simulink model "SistemaFunivia"  (R2023b)
settings: Solver=VariableStepAuto  StartTime=0.0  StopTime=100  FixedStep=1e-5
values from neighbouring files (symbols this model uses):
  dq_0 = [0; 0]    [Parametri.m]
  encoder_params = [r, encoder_accuracy, encoder_resolution, encoder_sample_rates]    [Parametri.m]
  encoder_resolution = 2*pi/1200    (= 0.00523598775598)    [Parametri.m]
  F_0 = 1500    [Parametri.m]
  L = 2.2    [Parametri.m]
  l = L - 1.2    (= 1)    [Parametri.m]
  laserd1_params = [laserd1_sample_rates, laserd1_resolution, laserd1_accuracy]    [Parametri.m]
  laserD_params = [laserD_sample_rates, laserD_resolution, laserD_accuracy]    [Parametri.m]
  min_sample_rates = max(sample_rates)    [Parametri.m]
  params = [m, c_a, J, L, l, h, r, g]    [Parametri.m]
  q_0 = [0; -pi/6]    [Parametri.m]
  q_hat_0 = [ dq_0(1) + normrnd(0, 0.1) ... (first row only)    [Parametri.m]
  R_k = diag([(laserD_accuracy/1000)^2, (laserd1_accuracy/1000)^2, (encoder_accuracy/encoder_sample_rates)^2])    [Parametri.m]
libraries: simulink x6, dspswit3 x1, embmathops x1
settings Model: Creator=lucag  LastModifiedBy=edoca

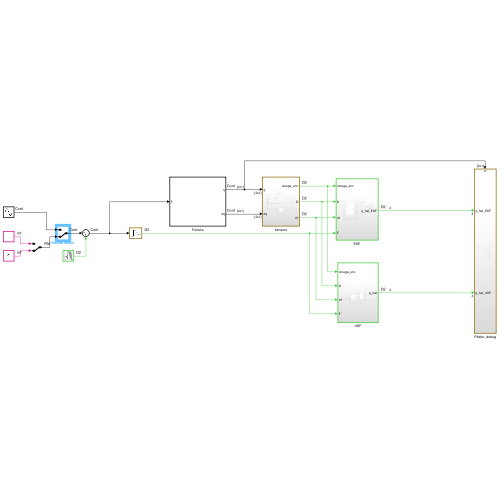
[thumbnail: Simulink's stored preview of the top-level diagram]
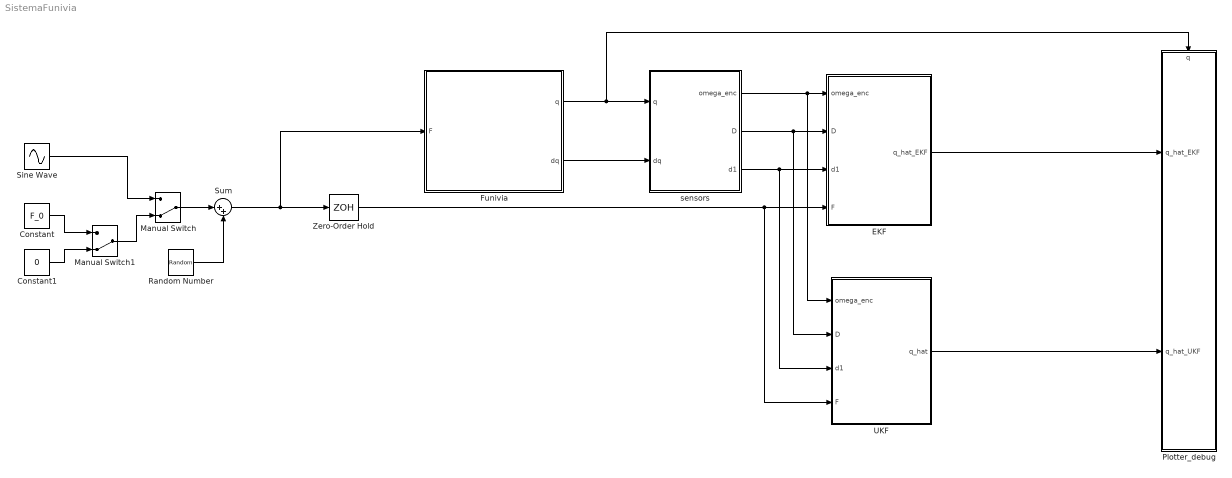
== system SistemaFunivia ==
  Constant : Constant  Value=F_0
  Constant1 : Constant  Value=0
  EKF : Subsystem
  Funivia : Subsystem
  Manual Switch : ManualSwitch  CurrentSetting=0
  Manual Switch1 : ManualSwitch  CurrentSetting=0
  Plotter_debug : Subsystem
      settings: PortSchema="{\"entries\":[{\"content\":{\"sides\":[{\"content\":{\"connectorIds\":[\"In1\",\"In2\"]},\"type\":\"ConnectorPlacement.EquallySpacedRectSide\",\"uuid\":\"d01a7d39-b326-48f3-bf6d-774b593ab054\"},{\"content\":{\"side\":\"RIGHT\"},\"type\":\"ConnectorPlacement.EquallySpacedRectSide\",\"uuid\":\"87cbfa34-b37b-41ae-99cb-fc2d681c6b8e\"},{\"content\":{\"connectorIds\":[\"In3\"],\"side\":\"TOP\"},\"type\":\"ConnectorPlacement.EquallySpacedRectSide\",\"uuid\":\"574a8c95-5b26-494e-b43d-53eefa443978\"}]},\"type\":\"ConnectorPlacement.EquallySpacedConnector\",\"uuid\":\"03fd7438-2859-47c7-88d3-b9f2a0aea320\"}],\"packageUris\":[\"http://schema.mathworks.com/mf0/Connector/R2020b\"],\"version\":\"1.0\"}"
  Random Number : RandomNumber  Variance=36  SampleTime=min_sample_rates
  Sine Wave : Sin  Amplitude=F_0  Frequency=pi/2  SampleTime=0
  Sum : Sum  Inputs=|++
  UKF : Subsystem
  Zero-Order Hold : ZeroOrderHold  SampleTime=min_sample_rates
  sensors : Subsystem
  wires:
  Sine Wave/1 -> Manual Switch/1
  Manual Switch/1 -> Sum/1
  Funivia/1(q) -> Plotter_debug/3(q), sensors/1(q)
  Funivia/2(dq) -> sensors/2(dq)
  sensors/1(omega_enc) -> UKF/1(omega_enc), EKF/1(omega_enc)
  sensors/2(D) -> EKF/2(D), UKF/2(D)
  sensors/3(d1) -> EKF/3(d1), UKF/3(d1)
  Zero-Order Hold/1 -> UKF/4(F), EKF/4(F)
  Sum/1 -> Zero-Order Hold/1, Funivia/1(F)
  Random Number/1 -> Sum/2
  EKF/1(q_hat_EKF) -> Plotter_debug/1(q_hat_EKF)
  UKF/1(q_hat) -> Plotter_debug/2(q_hat_UKF)
  Constant/1 -> Manual Switch1/1
  Constant1/1 -> Manual Switch1/2
  Manual Switch1/1 -> Manual Switch/2

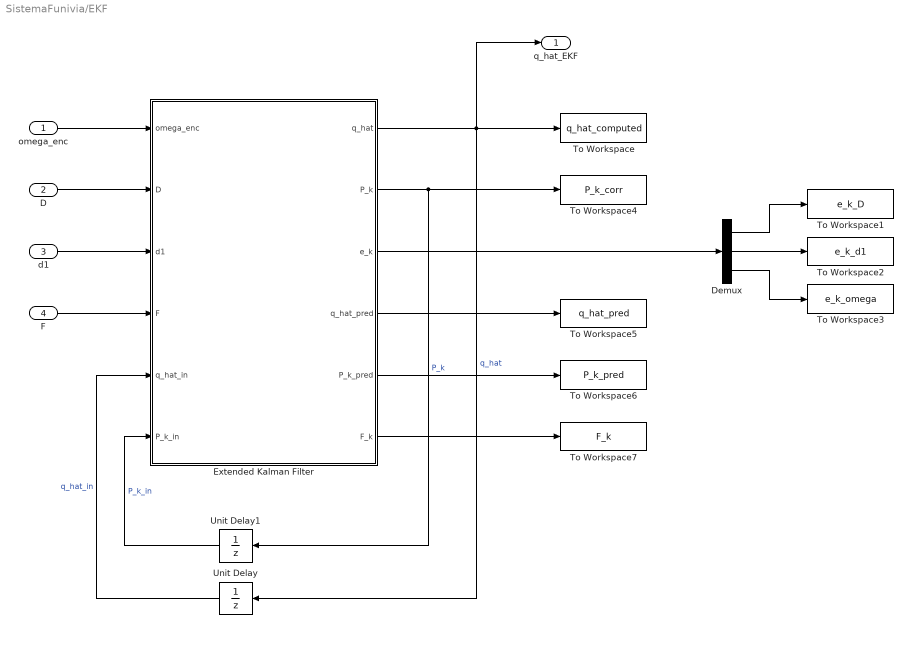
== system SistemaFunivia/EKF ==
  omega_enc : Inport
  D : Inport  Port=2
  d1 : Inport  Port=3
  F : Inport  Port=4
  Demux : Demux  Outputs=3
  Extended Kalman Filter : MATLAB Function  TreatAsAtomicUnit=on
  To Workspace : ToWorkspace  VariableName=q_hat_computed  SaveFormat=Timeseries  SampleTime=-1
  To Workspace1 : ToWorkspace  VariableName=e_k_D  SaveFormat=Timeseries  SampleTime=-1
  To Workspace2 : ToWorkspace  VariableName=e_k_d1  SaveFormat=Timeseries  SampleTime=-1
  To Workspace3 : ToWorkspace  VariableName=e_k_omega  SaveFormat=Timeseries  SampleTime=-1
  To Workspace4 : ToWorkspace  VariableName=P_k_corr  SaveFormat=Timeseries  SampleTime=-1
  To Workspace5 : ToWorkspace  VariableName=q_hat_pred  SaveFormat=Timeseries  SampleTime=-1
  To Workspace6 : ToWorkspace  VariableName=P_k_pred  SaveFormat=Timeseries  SampleTime=-1
  To Workspace7 : ToWorkspace  VariableName=F_k  SaveFormat=Timeseries  SampleTime=-1
  Unit Delay : UnitDelay  InitialCondition=q_hat_0  SampleTime=-1  HasFrameUpgradeWarning=on
  Unit Delay1 : UnitDelay  InitialCondition=eye(4)  SampleTime=-1  HasFrameUpgradeWarning=on
  q_hat_EKF : Outport
  wires:
  Extended Kalman Filter/2(P_k) -> Unit Delay1/1, To Workspace4/1  "P_k"
  omega_enc/1 -> Extended Kalman Filter/1(omega_enc)
  Unit Delay/1 -> Extended Kalman Filter/5(q_hat_in)  "q_hat_in"
  Extended Kalman Filter/1(q_hat) -> q_hat_EKF/1, To Workspace/1, Unit Delay/1  "q_hat"
  D/1 -> Extended Kalman Filter/2(D)
  F/1 -> Extended Kalman Filter/4(F)
  Unit Delay1/1 -> Extended Kalman Filter/6(P_k_in)  "P_k_in"
  d1/1 -> Extended Kalman Filter/3(d1)
  Extended Kalman Filter/3(e_k) -> Demux/1
  Demux/2 -> To Workspace2/1
  Demux/1 -> To Workspace1/1
  Demux/3 -> To Workspace3/1
  Extended Kalman Filter/4(q_hat_pred) -> To Workspace5/1
  Extended Kalman Filter/5(P_k_pred) -> To Workspace6/1
  Extended Kalman Filter/6(F_k) -> To Workspace7/1

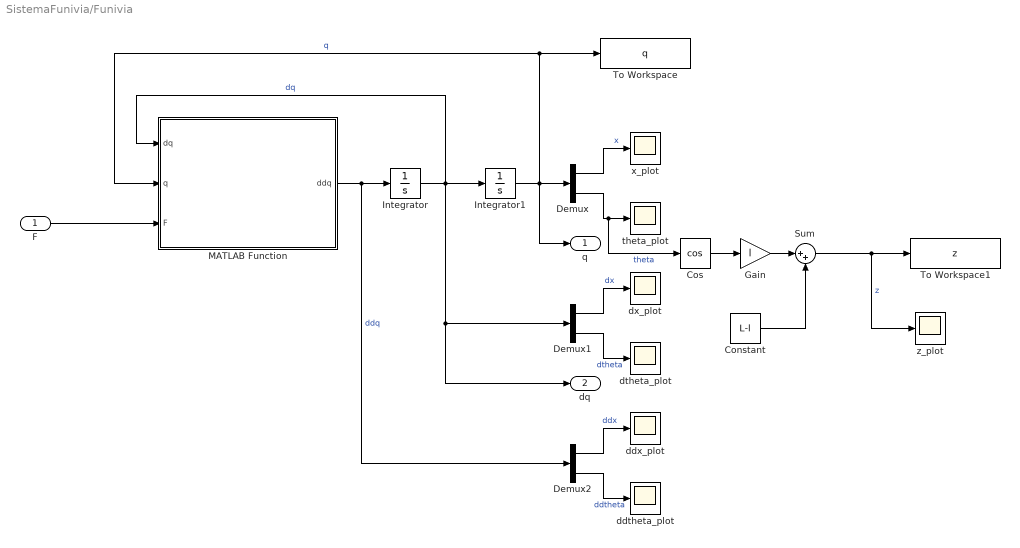
== system SistemaFunivia/Funivia ==
  F : Inport
  Constant : Constant  Value=L-l
  Cos : Trigonometry  Operator=cos
  Demux : Demux  Outputs=2
  Demux1 : Demux  Outputs=2
  Demux2 : Demux  Outputs=2
  Gain : Gain  Gain=l
  Integrator : Integrator  InitialCondition=dq_0
  Integrator1 : Integrator  InitialCondition=q_0
  MATLAB Function : MATLAB Function  TreatAsAtomicUnit=on
  Sum : Sum  Inputs=|++
  To Workspace : ToWorkspace  VariableName=q  SaveFormat=Timeseries  SampleTime=-1
  To Workspace1 : ToWorkspace  VariableName=z  SaveFormat=Timeseries  SampleTime=-1
  ddtheta_plot : Scope
  ddx_plot : Scope
  dtheta_plot : Scope
  dx_plot : Scope
  theta_plot : Scope
  x_plot : Scope
  z_plot : Scope
  q : Outport
  dq : Outport  Port=2
  wires:
  Demux/1 -> x_plot/1  "x"
  MATLAB Function/1(ddq) -> Demux2/1, Integrator/1  "ddq"
  Demux2/1 -> ddx_plot/1  "ddx"
  Integrator1/1 -> q/1, Demux/1, To Workspace/1, MATLAB Function/2(q)  "q"
  Integrator/1 -> dq/1, Demux1/1, MATLAB Function/1(dq), Integrator1/1  "dq"
  Demux2/2 -> ddtheta_plot/1  "ddtheta"
  Demux1/2 -> dtheta_plot/1  "dtheta"
  Demux/2 -> Cos/1, theta_plot/1  "theta"
  Demux1/1 -> dx_plot/1  "dx"
  F/1 -> MATLAB Function/3(F)
  Cos/1 -> Gain/1
  Gain/1 -> Sum/1
  Sum/1 -> z_plot/1, To Workspace1/1  "z"
  Constant/1 -> Sum/2

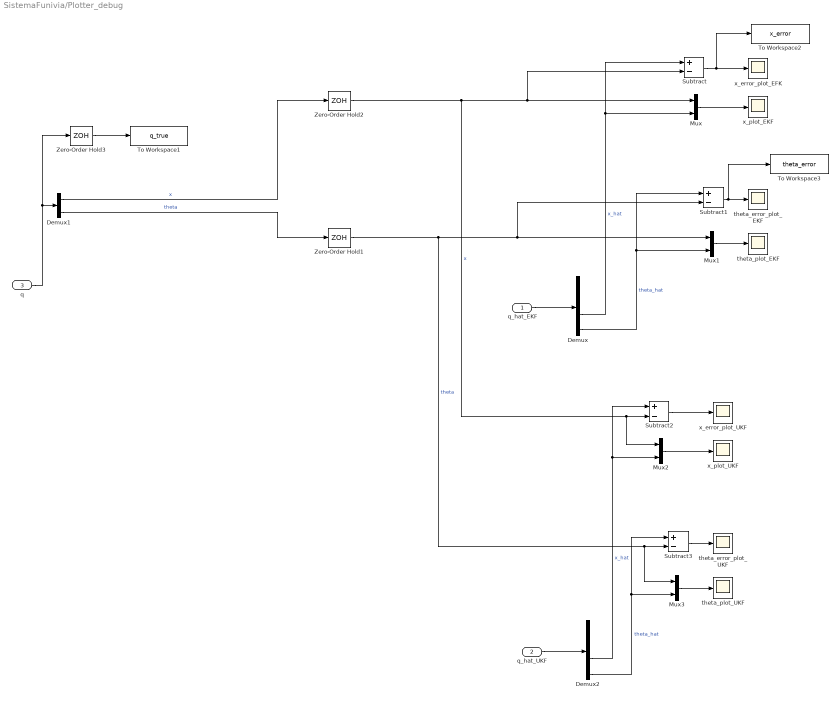
== system SistemaFunivia/Plotter_debug ==
  q_hat_EKF : Inport
  q_hat_UKF : Inport  Port=2
  q : Inport  Port=3
  Demux : Demux
  Demux1 : Demux  Outputs=2
  Demux2 : Demux
  Mux{,1..3} (4 alike) : Mux  Inputs=2
  Subtract{,1..3} (4 alike) : Sum  Inputs=+-
  To Workspace1 : ToWorkspace  VariableName=q_true  SaveFormat=Timeseries  SampleTime=-1
  To Workspace2 : ToWorkspace  VariableName=x_error  SaveFormat=Timeseries  SampleTime=-1
  To Workspace3 : ToWorkspace  VariableName=theta_error  SaveFormat=Timeseries  SampleTime=-1
  Zero-Order Hold1 : ZeroOrderHold  SampleTime=min_sample_rates
  Zero-Order Hold2 : ZeroOrderHold  SampleTime=min_sample_rates
  Zero-Order Hold3 : ZeroOrderHold  SampleTime=min_sample_rates
  theta_error_plot_EKF : Scope
  theta_error_plot_UKF : Scope
  theta_plot_EKF : Scope
  theta_plot_UKF : Scope
  x_error_plot_EFK : Scope
  x_error_plot_UKF : Scope
  x_plot_EKF : Scope
  x_plot_UKF : Scope
  wires:
  Mux/1 -> x_plot_EKF/1
  Demux/3 -> Mux/2, Subtract/1  "x_hat"
  q_hat_EKF/1 -> Demux/1
  Demux1/1 -> Zero-Order Hold2/1  "x"
  Zero-Order Hold3/1 -> To Workspace1/1
  Mux1/1 -> theta_plot_EKF/1
  Subtract1/1 -> To Workspace3/1, theta_error_plot_EKF/1
  Demux1/2 -> Zero-Order Hold1/1  "theta"
  q/1 -> Zero-Order Hold3/1, Demux1/1
  Demux/4 -> Subtract1/1, Mux1/2  "theta_hat"
  Subtract/1 -> To Workspace2/1, x_error_plot_EFK/1
  Demux2/4 -> Mux3/2, Subtract3/1  "theta_hat"
  Zero-Order Hold1/1 -> Mux1/1, Subtract1/2, Mux3/1, Subtract3/2  "theta"
  Subtract3/1 -> theta_error_plot_UKF/1
  Subtract2/1 -> x_error_plot_UKF/1
  Zero-Order Hold2/1 -> Mux/1, Subtract/2, Mux2/1, Subtract2/2  "x"
  Mux2/1 -> x_plot_UKF/1
  Demux2/3 -> Subtract2/1, Mux2/2  "x_hat"
  Mux3/1 -> theta_plot_UKF/1
  q_hat_UKF/1 -> Demux2/1

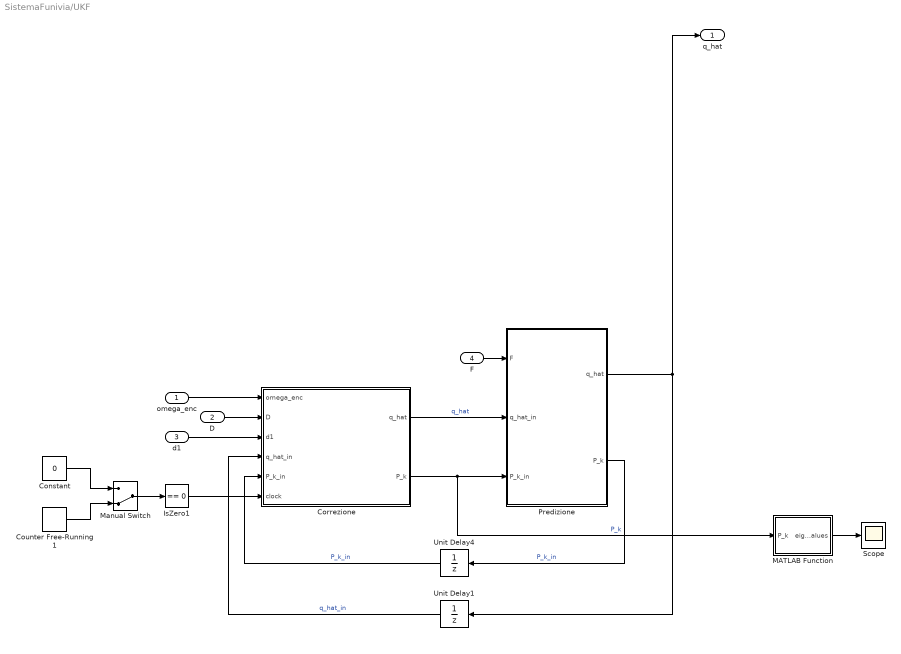
== system SistemaFunivia/UKF ==
  omega_enc : Inport
  D : Inport  Port=2
  d1 : Inport  Port=3
  F : Inport  Port=4
  Constant : Constant  Value=0
  Correzione : MATLAB Function  TreatAsAtomicUnit=on
  Counter Free-Running1 : simulink/Sources/Counter Free-Running  NumBits=1  tsamp=min_sample_rates
  IsZero1 : simulink/Logic and Bit Operations/Compare To Zero  relop===  OutDataTypeStr=boolean
      settings: LibrarySourceBlock=|
      | simulink/Quick Insert/Logic and Bit
      | Operations/IsZero
  MATLAB Function : MATLAB Function  TreatAsAtomicUnit=on
  Manual Switch : ManualSwitch  CurrentSetting=0
  Predizione : MATLAB Function  TreatAsAtomicUnit=on
  Scope : Scope
  Unit Delay1 : UnitDelay  InitialCondition=q_hat_0  SampleTime=-1  HasFrameUpgradeWarning=on
  Unit Delay4 : UnitDelay  InitialCondition=eye(4)  SampleTime=-1  HasFrameUpgradeWarning=on
  q_hat : Outport
  wires:
  Correzione/1(q_hat) -> Predizione/2(q_hat_in)  "q_hat"
  Correzione/2(P_k) -> MATLAB Function/1(P_k), Predizione/3(P_k_in)  "P_k"
  Unit Delay1/1 -> Correzione/4(q_hat_in)  "q_hat_in"
  Predizione/2(P_k) -> Unit Delay4/1  "P_k_in"
  Unit Delay4/1 -> Correzione/5(P_k_in)  "P_k_in"
  Predizione/1(q_hat) -> Unit Delay1/1, q_hat/1
  IsZero1/1 -> Correzione/6(clock)
  MATLAB Function/1(eigenvalues) -> Scope/1
  F/1 -> Predizione/1(F)
  omega_enc/1 -> Correzione/1(omega_enc)
  D/1 -> Correzione/2(D)
  d1/1 -> Correzione/3(d1)
  Manual Switch/1 -> IsZero1/1
  Constant/1 -> Manual Switch/1
  Counter Free-Running1/1 -> Manual Switch/2

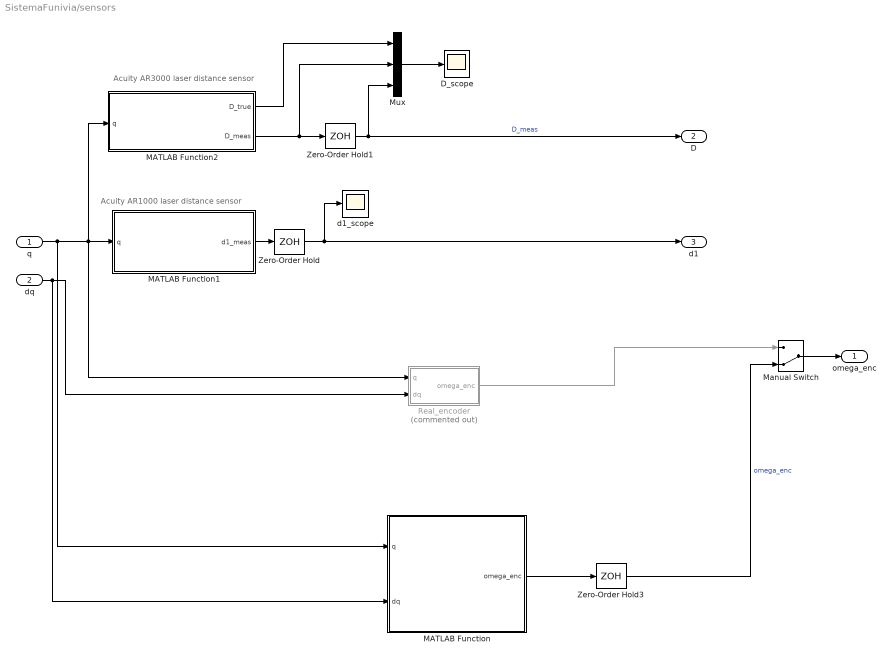
== system SistemaFunivia/sensors ==
  note: Acuity AR1000 laser distance sensor
  note: Acuity AR3000 laser distance sensor
  q : Inport
  dq : Inport  Port=2
  D_scope : Scope
  MATLAB Function : MATLAB Function  TreatAsAtomicUnit=on
  MATLAB Function1 : MATLAB Function  TreatAsAtomicUnit=on
  MATLAB Function2 : MATLAB Function  TreatAsAtomicUnit=on  SystemSampleTime=1/100
  Manual Switch : ManualSwitch  CurrentSetting=0
  Mux : Mux  Inputs=3
  Real_encoder : Subsystem  Commented=on
  Zero-Order Hold : ZeroOrderHold  SampleTime=min_sample_rates
  Zero-Order Hold1 : ZeroOrderHold  SampleTime=min_sample_rates
  Zero-Order Hold3 : ZeroOrderHold  SampleTime=min_sample_rates
  d1_scope : Scope
  omega_enc : Outport
  D : Outport  Port=2
  d1 : Outport  Port=3
  wires:
  Zero-Order Hold/1 -> d1/1, d1_scope/1
  Zero-Order Hold1/1 -> D/1, Mux/3  "D_meas"
  Mux/1 -> D_scope/1
  q/1 -> MATLAB Function/1(q), Real_encoder/1(q), MATLAB Function2/1(q), MATLAB Function1/1(q)
  MATLAB Function2/2(D_meas) -> Mux/2, Zero-Order Hold1/1
  MATLAB Function2/1(D_true) -> Mux/1
  MATLAB Function1/1(d1_meas) -> Zero-Order Hold/1
  dq/1 -> Real_encoder/2(dq), MATLAB Function/2(dq)
  Manual Switch/1 -> omega_enc/1
  MATLAB Function/1(omega_enc) -> Zero-Order Hold3/1
  Zero-Order Hold3/1 -> Manual Switch/2  "omega_enc"
  Real_encoder/1(omega_enc) -> Manual Switch/1

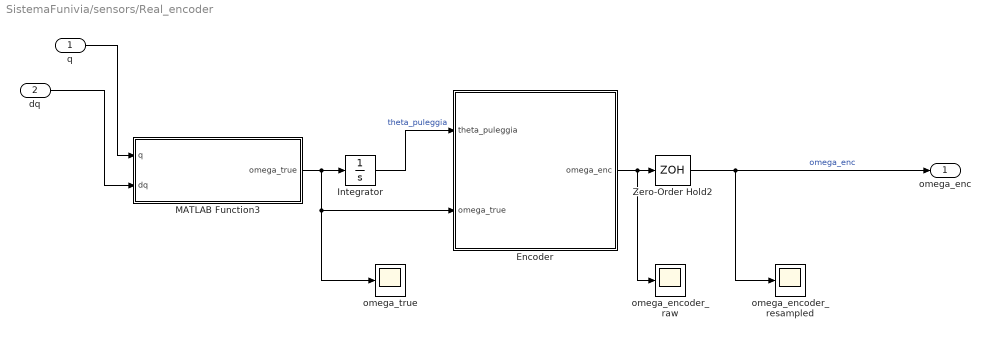
== system SistemaFunivia/sensors/Real_encoder ==
  q : Inport
  dq : Inport  Port=2
  Encoder : Subsystem
  Integrator : Integrator
  MATLAB Function3 : MATLAB Function  TreatAsAtomicUnit=on
  Zero-Order Hold2 : ZeroOrderHold  SampleTime=min_sample_rates
  omega_encoder_raw : Scope
  omega_encoder_resampled : Scope
  omega_true : Scope
  omega_enc : Outport
  wires:
  q/1 -> MATLAB Function3/1(q)
  Encoder/1(omega_enc) -> omega_encoder_raw/1, Zero-Order Hold2/1
  MATLAB Function3/1(omega_true) -> Encoder/2(omega_true), omega_true/1, Integrator/1
  dq/1 -> MATLAB Function3/2(dq)
  Integrator/1 -> Encoder/1(theta_puleggia)  "theta_puleggia"
  Zero-Order Hold2/1 -> omega_enc/1, omega_encoder_resampled/1  "omega_enc"

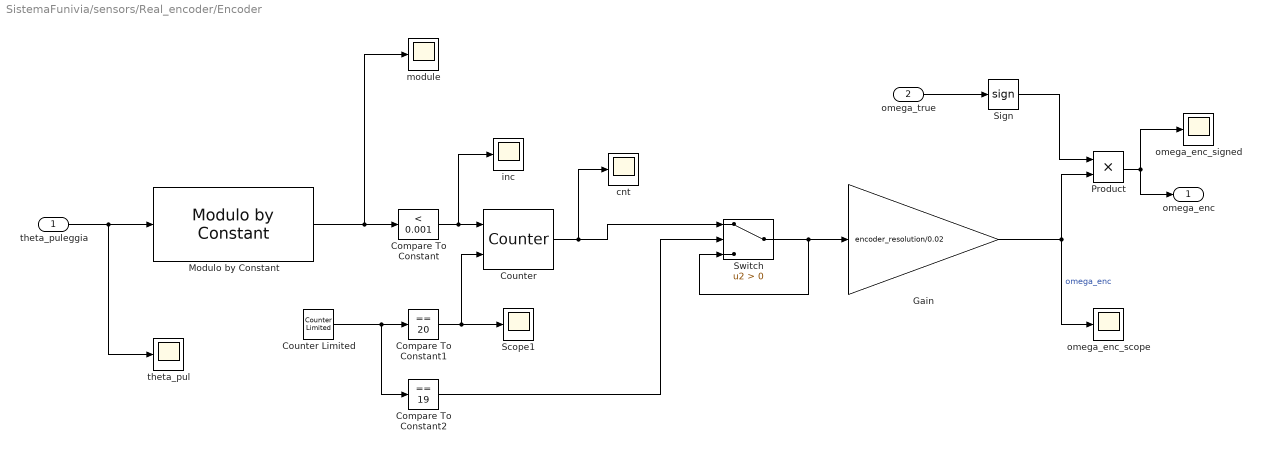
== system SistemaFunivia/sensors/Real_encoder/Encoder ==
  theta_puleggia : Inport
  omega_true : Inport  Port=2
  Compare To Constant : simulink/Logic and Bit Operations/Compare To Constant  relop=<  const=0.001  OutDataTypeStr=boolean
  Compare To Constant1 : simulink/Logic and Bit Operations/Compare To Constant  relop===  const=20  OutDataTypeStr=boolean
  Compare To Constant2 : simulink/Logic and Bit Operations/Compare To Constant  relop===  const=19  OutDataTypeStr=boolean
  Counter : dspswit3/Counter  Direction=Up  CountEvent=Rising edge  CounterSize=User defined  MaxCount=65535  InitialCount=0  Output=Count  HitValue=32  ResetInput=on  SamplesPerFrame=1  Ts=1  CntDtype=double  HitDtype=Logical
  Counter Limited : simulink/Sources/Counter Limited  uplimit=20  tsamp=0.001
  Gain : Gain  Gain=encoder_resolution/0.02
  Modulo by Constant : embmathops/Modulo by Constant  Denominator=encoder_resolution  SimulateUsing=Code generation
      settings: LibrarySourceBlock=embeddedMathLib/Modulo by Constant
  Product : Product
  Scope1 : Scope
  Sign : Signum
  Switch : Switch  Criteria=u2 > Threshold  SaturateOnIntegerOverflow=off  InputSameDT=off
  cnt : Scope
  inc : Scope
  module : Scope
  omega_enc_scope : Scope
  omega_enc_signed : Scope
  theta_pul : Scope
  omega_enc : Outport
  wires:
  Counter/1 -> cnt/1, Switch/1
  Switch/1 -> Switch/3, Gain/1
  Modulo by Constant/1 -> module/1, Compare To Constant/1
  Counter Limited/1 -> Compare To Constant2/1, Compare To Constant1/1
  Compare To Constant1/1 -> Scope1/1, Counter/2
  Gain/1 -> Product/2, omega_enc_scope/1  "omega_enc"
  Compare To Constant2/1 -> Switch/2
  Compare To Constant/1 -> inc/1, Counter/1
  theta_puleggia/1 -> Modulo by Constant/1, theta_pul/1
  omega_true/1 -> Sign/1
  Product/1 -> omega_enc_signed/1, omega_enc/1
  Sign/1 -> Product/1

== matlab function SistemaFunivia/UKF/Predizione ==
  settings: sampleTime=min_sample_rates
  data: F input; q_hat_in input; q_hat output; P_k_in input; P_k output; params parameter; min_sample_rates parameter
function [q_hat, P_k] = prediction(F, q_hat_in, P_k_in, params, min_sample_rates)
    m = params(1);
    c_a = params(2);
    J = params(3);
    
    L = params(4);
    l = params(5);
    h = params(6);
    r = params(7);
    
    g = params(8);

    dev_std = 6;
    Q_k = dev_std^2;

    dt = min_sample_rates;
    

    x_UT = [q_hat_in; 0]; %[5x1]
    sigma = blkdiag(P_k_in, Q_k); %[5x5]

    alpha = 1;            % not scaled
    beta = 2;             % optimum for the Gaussian case
    kappa = 0;

    enne = size(x_UT,1); % =5

    lambda = alpha^2*(enne + kappa) - enne;

    % compute weights
    wc = zeros(1, 2*enne+1);   %[1x11]

    w0 = lambda/(lambda + enne);
    wc(1) = w0 + 1 - alpha^2 + beta;
    wc(2:2*enne+1) = 1/2/(enne+lambda);

    wm = wc;%[1x11]
    wm(1) = w0;

    % factorise covariance matrix
    [U,S,~] = svd(sigma);
    Gamma = U*sqrtm(S);
    
    % generate 2n+1 sigma points
    sigma_points = [x_UT, zeros(5,10)];
    for i = 1:size(Gamma,2)
        sigma_points(:,i+1)      = x_UT + sqrt(enne+lambda)*real(Gamma(:,i));
        sigma_points(:,i+1+enne) = x_UT - sqrt(enne+lambda)*real(Gamma(:,i));
    end
    
    propagated_sigma_points = zeros(4, size(sigma_points,2)); %[4x11]

    for i = 1:size(sigma_points,2)
        propagated_sigma_points(1,i) = sigma_points(1,i) + dt*(-(c_a/m)*(sigma_points(1,i)-(l+r)*sigma_points(2,i)*cos(sigma_points(4,i)))+ (1/m)*F);
        propagated_sigma_points(2,i) = sigma_points(2,i) + dt*(-(m*g*(l+r)/J)*(sin(sigma_points(4,i))) + (c_a*(l+r)/J)*(sigma_points(1,i) - (l+r)*sigma_points(2,i)*cos(sigma_points(4,i)) - F*(L/J)*cos(sigma_points(4,i))));
        propagated_sigma_points(3,i) = sigma_points(3,i) + dt*sigma_points(1,i);
        propagated_sigma_points(4,i) = sigma_points(4,i) + dt*sigma_points(2,i);
    end

    % compute propagated mean
    propagated_mean = propagated_sigma_points*wm'; % [4x11] * [11x1] = [4x1]
    
    % Set dimension for propagated_tilde [4x11]
    propagated_tilde = propagated_sigma_points - propagated_mean;

    % %propagated ~ ( x~ = x - x_mean )
    % for i = 1:size(propagated_sigma_points,2)
    %     propagated_tilde(:,i) = propagated_sigma_points(:,i) - propagated_mean;
    % end

    % compute virtual measurements second order
    propagated_cov = zeros(4,4);

    for i = 1:size(sigma_points,2)
        propagated_cov = propagated_cov + wc(i)*propagated_tilde(:,i)*propagated_tilde(:,i)';
    end

    q_hat = propagated_mean;
    P_k = propagated_cov;

== matlab function SistemaFunivia/UKF/Correzione ==
  settings: sampleTime=min_sample_rates
  data: omega_enc input; D input; d1 input; q_hat_in input; q_hat output; P_k_in input; P_k output; params parameter; R_k parameter; clock input
function [q_hat, P_k] = correction(omega_enc, D, d1, q_hat_in, P_k_in, params, R_k, clock)

if(clock == 1)
    L = params(4);
    l = params(5);
    h = params(6);
    r = params(7);

    alpha = 1;            % not scaled
    beta = 2;             % optimum for the Gaussian case
    kappa = 0;

    enne = size(q_hat_in,1); % = 4

    lambda = alpha^2*(enne + kappa) - enne;

    % compute weights
    wc = zeros(1, 2*enne+1);   %[1x9]

    w0 = lambda/(lambda + enne);
    wc(1) = w0 + 1 - alpha^2 + beta;
    wc(2:2*enne+1) = 1/2/(enne+lambda);

    wm = wc; %[1x9]
    wm(1) = w0;

    % factorise covariance matrix
    [U,S,~] = svd(P_k_in);
    Gamma = U*sqrtm(S);
    
    % generate 2n+1 sigma points
    sigma_points = [q_hat_in, zeros(4,8)];
    for i = 1:size(Gamma,2)
        sigma_points(:,i+1)      = q_hat_in + sqrt(enne+lambda)*real(Gamma(:,i));
        sigma_points(:,i+1+enne) = q_hat_in - sqrt(enne+lambda)*real(Gamma(:,i));
    end

    propagated_sigma_points = zeros(3, size(sigma_points,2)); %[3x9]

    % apply function h to the 2n+1 sigma points
    for i = 1:size(sigma_points,2)
        propagated_sigma_points(1,i) = sigma_points(3, i) + (l + r)*sin(sigma_points(4, i));
        propagated_sigma_points(2,i) = (L + h) * cos(sigma_points(4, i));
        propagated_sigma_points(3,i) = (sigma_points(1, i) - (l + r)*sigma_points(2, i)*cos(sigma_points(4, i))) / r;
    end
    
    % Propagated mean of measurements
    propagated_meas_mean = propagated_sigma_points*wm'; % [3x9] * [9x1] = [3x1]

    % Propagated tilde of measurements
    propagated_meas_tilde = propagated_sigma_points - propagated_meas_mean; % [3x9] - [3x1] = [3x9]  (how matlab works)
    
    % Matrix Covariance of measurements
    meas_cov = zeros(3, 3);
    cross_cov = zeros(4, 3); 

    for i = 1:size(sigma_points,2)
        meas_cov = meas_cov + wc(i) * propagated_meas_tilde(:,i) * propagated_meas_tilde(:,i)';
        cross_cov = cross_cov + wc(i) * (sigma_points(:,i) - q_hat_in) * propagated_meas_tilde(:,i)'; %    wc * (x~ * y~)
    end

    % Fine algoritmo UT e inzio calcolo matrici per correzione
    
    y = [D; d1; omega_enc];
    y_hat = propagated_meas_mean;

    e_k = y - y_hat;
    S_k = meas_cov + R_k;
    L_k = cross_cov * S_k^(-1);
    
    % Matrici per forma di Joseph
    H_k = cross_cov' / (P_k_in);
    K_k = cross_cov / meas_cov;

    q_hat = q_hat_in + L_k * e_k;
    P_k = (eye(4) - K_k * H_k) * P_k_in * (eye(4) - K_k * H_k)' + K_k * R_k * K_k';
    % P_k = P_k_in - L_k * S_k * L_k';
else
    q_hat = q_hat_in;
    P_k = P_k_in;

end

== matlab function SistemaFunivia/UKF/MATLAB Function ==
  data: P_k input; eigenvalues output
function eigenvalues = fcn(P_k)

    eigenvalues = eig(P_k);

end

== matlab function SistemaFunivia/sensors/MATLAB Function2 ==
  settings: updateMethod=DISCRETE  sampleTime=laserD_sample_rates
  data: D_true output; D_meas output; q input; params parameter; laserD_params parameter
function [D_true, D_meas] = Sensore_Laser_D(q, params, laserD_params)
    laserD_accuracy = laserD_params(3); %[mm]
    l = params(5)*1000; %[mm]
    r = params(7)*1000; %[mm]

    x = q(1)*1000; %[mm]
    theta = q(2);

    D_true = x + (l+r)*sin(theta);  % [mm]
    noise = normrnd(0, laserD_accuracy);  

    D_meas = D_true + noise;   % convert the data params from meters to mm, because the noise is in mm
    D_meas = round(D_meas)/1000;
end

== matlab function SistemaFunivia/Funivia/MATLAB Function ==
  settings: updateMethod=CONTINUOUS
  data: dq input; ddq output; q input; F input; params_incert parameter
function ddq = ModelloDinamicoFunivia(dq, q, F, params_incert)
    % params = [m, c_a, J, L, l, h, r, g];
    %           1, 2,   3, 4, 5, 6, 7 ,8

    % Variabili di Stato %
    dx = dq(1);
    dtheta = dq(2);

    x = q(1);
    theta = q(2);
   
    % Parametri fisici (con incertezza)
    m = params_incert(1);
    c_a = params_incert(2);
    J = params_incert(3);

    L = params_incert(4);
    l = params_incert(5);
    h = params_incert(6);
    r = params_incert(7);

    g = params_incert(8);

    % Equazioni del modello fisico %
    ddx = -c_a/m * (dx - (l + r)*dtheta*cos(theta)) + F/m;
    ddtheta = -m*g*(l + r)/J * sin(theta) + c_a*(l + r)/J * (dx - (l + r)*dtheta*cos(theta)) - F*L/J * cos(theta);

    ddq = [ddx; ddtheta];

end

== matlab function SistemaFunivia/sensors/MATLAB Function1 ==
  settings: updateMethod=DISCRETE  sampleTime=laserd1_sample_rates
  data: d1_meas output; q input; params parameter; laserd1_params parameter
function d1_meas = Sensore_Laser_d1(q, params, laserd1_params)
    
    L = params(4);
    h = params(6);

    laser_accuracy = laserd1_params(3);

    theta = q(2);
    
    d1_true = (L + h) * 1000 * cos(theta);    % [mm]
    noise = normrnd(0, laser_accuracy);

    d1_meas = d1_true + noise;
    d1_meas = round(d1_meas) / 1000;    % to meters

end

== matlab function SistemaFunivia/sensors/Real_encoder/MATLAB Function3 ==
  settings: updateMethod=CONTINUOUS  sampleTime=encoder_sample_rates
  data: omega_true output; q input; params parameter; encoder_params parameter; dq input
function omega_true = puleggia(q, params, encoder_params, dq)
    
    l = params(5); % [m]
    r = encoder_params(1); % [m]

    theta = q(2); % [rad]

    dx = dq(1); % [m/s]
    dtheta = dq(2); % [rad/s]

    v_c = dx - l*dtheta*cos(theta); %equation
    
    omega_true = v_c/r;    % [rad/s]
    % noise = normrnd(0, encoder_accuracy/3);
    % 
    % omega_meas = omega_true + noise;
    % omega = round(omega_meas);

end

== matlab function SistemaFunivia/EKF/Extended Kalman Filter ==
  settings: updateMethod=DISCRETE  sampleTime=min_sample_rates
  data: omega_enc input; D input; d1 input; params parameter; F input; min_sample_rates parameter; q_hat output; P_k output; R_k parameter; q_hat_in input; P_k_in input; e_k output; q_hat_pred output; P_k_pred output; F_k output
function [q_hat, P_k, e_k, q_hat_pred, P_k_pred, F_k] = EKF(omega_enc, D, d1, params, F, min_sample_rates, R_k, q_hat_in, P_k_in)

% parametri = [m, c_a, J, L, l, h, r, g];

m = params(1);         
c_a = params(2);
J = params(3);

L = params(4);
l = params(5);
h = params(6);
r = params(7);

g = params(8);

q1 = q_hat_in(1);   % x_dot
q2 = q_hat_in(2);   % theta_dot
q3 = q_hat_in(3);   % x
q4 = q_hat_in(4);   % theta

%% Predizione

% Linearizzazione sistema dinamico T.C.
F_k = [-c_a/m,          (c_a/m)*(l+r)*cos(q4),      0,      -(c_a/m)*(l+r)*q2*sin(q4);
        c_a*(l+r)/J,    -(c_a*(l+r)^2/J)*cos(q4),   0,      -(m*g*(l+r)/J)*cos(q4) + (c_a*(l+r)^2/J)*q2*sin(q4) + F*(L/J)*sin(q4);
        1,              0,                          0,      0;
        0,              1,                          0,      0];

D_k = [1/m;
      -(L/J)*cos(q4);
      0;
      0];

% Conversione TC a TD:    q_dot  =>  (q_k+1 - q_k)/dT = F_k * q_k + D_k * F
F_k = min_sample_rates .* F_k + eye(4);  
D_k = min_sample_rates .* D_k;

% Definizione matrice di varianza del rumore in ingresso 
dev_std = 6;
Q_k = dev_std^2;

% Algoritmo di Predizione
P_k = F_k * P_k_in * F_k' + D_k * Q_k * D_k';
q_hat = q_hat_in + min_sample_rates .* [-c_a/m * (q1 - (l + r)*q2*cos(q4)) + F/m;
                                        -m*g*(l + r)/J * sin(q4) + c_a*(l + r)/J * (q1 - (l + r)*q2*cos(q4)) - F*L/J * cos(q4);
                                        q1;
                                        q2];

q_hat_pred = q_hat;
P_k_pred = P_k;

%% Correzione

% Misura dei sensori
y_k = [D;
       d1;
       omega_enc];

% Dinamica uscita sistema 
h_k = [q3 + (l+r)*sin(q4);
       (L+h)*cos(q4);
       (1/r)*(q1 - (l+r)*q2*cos(q4))];

% Linearizzazione dinamica di uscita del sistema
H_k = [0,           0,                      1,      (l+r)*cos(q4);
       0,           0,                      0,      -(L+h)*sin(q4);
       1/r,         -((l+r)/r)*cos(q4),     0,      ((l+r)/r)*q2*sin(q4)];

% Definizione matrice di varianza del rumore sulla misura
M_k = eye(3);   % Ipotesi: rumore gaussiano equamente distribuito per ogni misura dei sensori


% Calcolo Innovazione, Covarianza Innovazione, Guadagno di Correzione
e_k = y_k - h_k;
S_k = H_k * P_k * H_k' + M_k * R_k * M_k';
L_k = P_k * H_k' * S_k^(-1);

% Algoritmo di correzione della stima
q_hat = q_hat + L_k * e_k;
P_k = (eye(4) - L_k * H_k)*P_k*(eye(4) - L_k*H_k)' + L_k * M_k * R_k * M_k' * L_k'; % Uso della forma di Joshep

% P_k = P_k - L_k * S_k * L_k';

end

== matlab function SistemaFunivia/sensors/MATLAB Function ==
  settings: updateMethod=DISCRETE  sampleTime=encoder_sample_rates
  data: q input; dq input; omega_enc output; params parameter; encoder_params parameter
function omega_enc = encoder(q, dq, params, encoder_params)
    % params = [m, c_a, J, L, l, h, r, g];
    %           1, 2,   3, 4, 5, 6, 7 ,8
    l = params(5);
    r = params(7);
    encoder_accuracy = encoder_params(2);
    encoder_sample_rates = encoder_params(4);

    theta = q(2);
    dtheta = dq(2);
    dx = dq(1);
    
    omega_true = (dx - (l+r)*dtheta*cos(theta))/r;    % [rad/s]
    noise = normrnd(0, encoder_accuracy/(encoder_sample_rates));

    omega_enc = omega_true + noise;

end
